simulink model "ControlBA"  (R2023b)
settings: Solver=VariableStepAuto  StartTime=0.0  StopTime=10.0  RelTol=1e-3
settings Model: Creator=Usuario_UMA  LastModifiedBy=Usuario_UMA

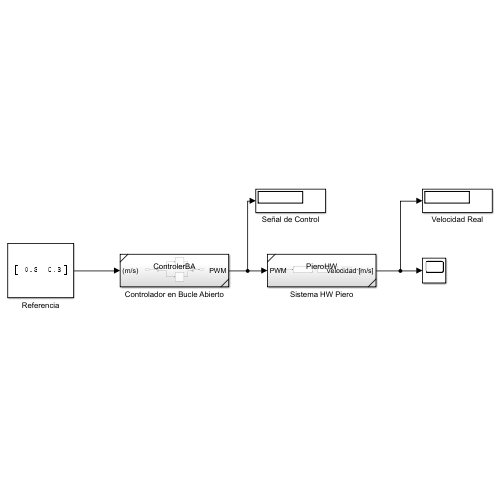
[thumbnail: Simulink's stored preview of the top-level diagram]
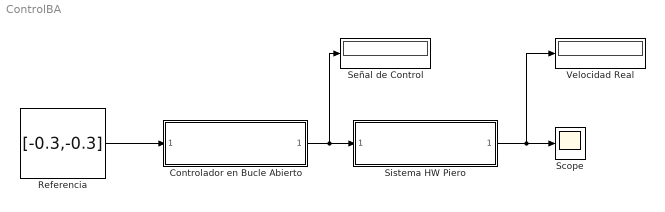
== system ControlBA ==
  Controlador en Bucle Abierto : Subsystem  ReferencedSubsystem=ControlerBA
  Referencia : Constant  Value=[-0.3,-0.3]
  Scope : Scope
  Señal de Control : Display
  Sistema HW Piero : Subsystem  ReferencedSubsystem=PieroHW
  Velocidad Real : Display
  wires:
  Controlador en Bucle Abierto/1 -> Señal de Control/1, Sistema HW Piero/1
  Referencia/1 -> Controlador en Bucle Abierto/1
  Sistema HW Piero/1 -> Velocidad Real/1, Scope/1
